simulink model "Three_Phase_Full_Wave_Uncontrolled_Rectifier"  (R2017b)
settings: Solver=VariableStepAuto  StartTime=0.0  StopTime=1.0  MaxStep=1e-4  RelTol=1e-3
libraries: powerlib x24, powerlib_meascontrol x5
settings Model: Creator=DELL  LastModifiedBy=DELL

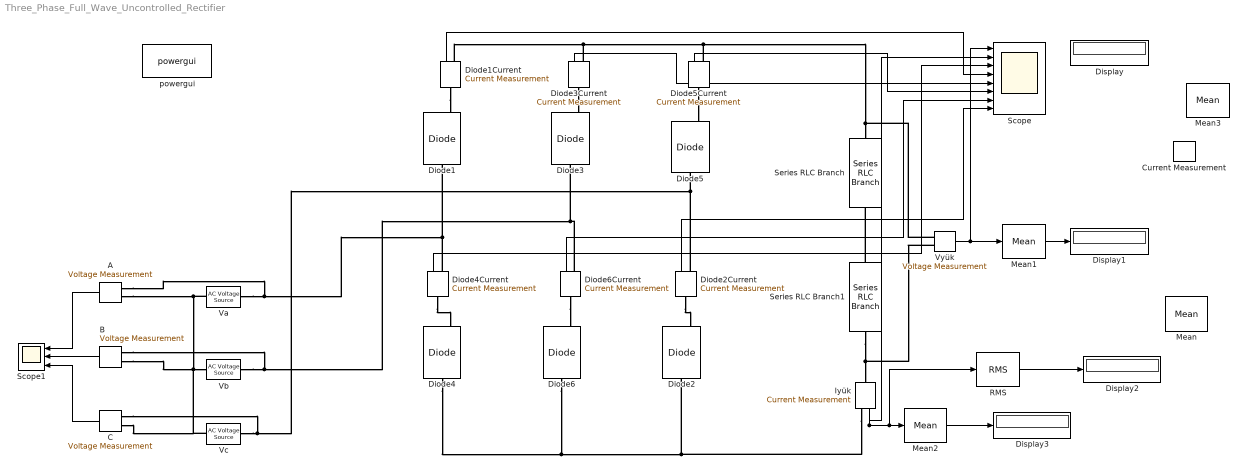
== system Three_Phase_Full_Wave_Uncontrolled_Rectifier ==
  A : powerlib/Measurements/Voltage Measurement  PhasorSimulation=off  OutputType=Complex  PSBequivalent=0
  B : powerlib/Measurements/Voltage Measurement  PhasorSimulation=off  OutputType=Complex  PSBequivalent=0
  C : powerlib/Measurements/Voltage Measurement  PhasorSimulation=off  OutputType=Complex  PSBequivalent=0
  Current Measurement : powerlib/Measurements/Current Measurement  PhasorSimulation=off  OutputType=Complex  PSBequivalent=0
  Diode{1..6} (6 alike) : powerlib/Power Electronics/Diode  Ron=0.001  Lon=0  Vf=0.8  IC=0  UseSnubber=0  Rs=500  Cs=250e-9  Measurements=on
  Diode1Current : powerlib/Measurements/Current Measurement  PhasorSimulation=off  OutputType=Complex  PSBequivalent=0
  Diode2Current : powerlib/Measurements/Current Measurement  PhasorSimulation=off  OutputType=Complex  PSBequivalent=0
  Diode3Current : powerlib/Measurements/Current Measurement  PhasorSimulation=off  OutputType=Complex  PSBequivalent=0
  Diode4Current : powerlib/Measurements/Current Measurement  PhasorSimulation=off  OutputType=Complex  PSBequivalent=0
  Diode5Current : powerlib/Measurements/Current Measurement  PhasorSimulation=off  OutputType=Complex  PSBequivalent=0
  Diode6Current : powerlib/Measurements/Current Measurement  PhasorSimulation=off  OutputType=Complex  PSBequivalent=0
  Display{,1..3} (4 alike) : Display
  Iyük : powerlib/Measurements/Current Measurement  PhasorSimulation=off  OutputType=Complex  PSBequivalent=0
  Mean : powerlib_meascontrol/Measurements/Mean  Freq=60  Vinit=0  Ts=0
  Mean1 : powerlib_meascontrol/Measurements/Mean  Freq=50  Vinit=0  Ts=0
  Mean2 : powerlib_meascontrol/Measurements/Mean  Freq=50  Vinit=0  Ts=0
  Mean3 : powerlib_meascontrol/Measurements/Mean  Freq=60  Vinit=0  Ts=0
  RMS : powerlib_meascontrol/Measurements/RMS  TrueRMS=on  Freq=50  RMSInit=120  Ts=0
  Scope : Scope  NumInputPorts=8
  Scope1 : Scope  NumInputPorts=3
  Series RLC Branch : powerlib/Elements/Series RLC Branch  LConnTagsString=__new0  RConnTagsString=__new0  BranchType=L  Resistance=1  Inductance=20e-3  SetiL0=off  InitialCurrent=0  Capacitance=1e-6  Setx0=off  InitialVoltage=0  Measurements=None
  Series RLC Branch1 : powerlib/Elements/Series RLC Branch  LConnTagsString=__new0  RConnTagsString=__new0  BranchType=R  Resistance=10  Inductance=1e-3  SetiL0=off  InitialCurrent=0  Capacitance=1e-6  Setx0=off  InitialVoltage=0  Measurements=None
  Va : powerlib/Electrical Sources/AC Voltage Source  Amplitude=220*(2^0.5)  Phase=0  Frequency=50  SampleTime=0  Measurements=None  BusType=swing  Pref=10e3  Qref=0  Qmin=-inf  Qmax=+inf
  Vb : powerlib/Electrical Sources/AC Voltage Source  Amplitude=220*(2^0.5)  Phase=-120  Frequency=50  SampleTime=0  Measurements=None  BusType=swing  Pref=10e3  Qref=0  Qmin=-inf  Qmax=+inf
  Vc : powerlib/Electrical Sources/AC Voltage Source  Amplitude=220*(2^0.5)  Phase=120  Frequency=50  SampleTime=0  Measurements=None  BusType=swing  Pref=10e3  Qref=0  Qmin=-inf  Qmax=+inf
  Vyük : powerlib/Measurements/Voltage Measurement  PhasorSimulation=off  OutputType=Complex  PSBequivalent=0
  powergui : powerlib/powergui  Priority=1  SimulationMode=Continuous  SampleTime=50e-6  frequency=60  Iterations=50  frequencyindice=50  Pbase=100e6  ErrMax=1e-4  UnitsV=kV  UnitsW=MW  buscounter=0  FunctionMessages=off  echomessages=off  EnableUseOfTLC=off  CurrentSourceSwitches=off  DisableSnubberDevices=off  DisableRonSwitches=off  DisableVfSwitches=off  DisplayEquations=off  SolverType=Tustin/Backward Euler (TBE)  Interpol=off  ExternalGateDelay=off  methode=off  Ts=100  x0status=blocks  SPID=on  SwTol=0  HookPort=off  RestoreLinks=warning  ResistiveCurrentMeasurement=off  Frange=[0:2:500]  Ylog=off  Xlog=on  ShowGrid=off  save=off  variable=ZData  structure=0  ZoomFFT=off  StartTime=0.0  cycles=1  DisplayStyle=1  fundamental=60  FreqAxis=off  MaxFrequency=1000  frequencyindicesteady=1  RmsSteady=1  display=off
  wires:
  A/1 -> Scope1/1
  B/1 -> Scope1/2
  C/1 -> Scope1/3
  Iyük/1 -> RMS/1, Mean2/1, Scope/2
  Vyük/1 -> Scope/1, Mean1/1
  Mean2/1 -> Display3/1
  RMS/1 -> Display2/1
  Mean1/1 -> Display1/1
  Diode5Current/1 -> Scope/6
  Diode4Current/1 -> Scope/3
  Diode1Current/1 -> Scope/4
  Diode3Current/1 -> Scope/5
  Diode6Current/1 -> Scope/7
  Diode2Current/1 -> Scope/8
  connections:
  Va/RConn1 -- A/LConn1 -- Diode4Current/RConn1 -- Diode1/LConn1
  Diode3Current/RConn1 -- Diode5Current/RConn1 -- Vyük/LConn1 -- Series RLC Branch/RConn1 -- Diode1Current/RConn1
  Series RLC Branch1/RConn1 -- Series RLC Branch/LConn1
  Diode6/LConn1 -- Iyük/RConn1 -- Diode2/LConn1 -- Diode4/LConn1
  Vb/RConn1 -- B/LConn1 -- Diode3/LConn1 -- Diode6Current/RConn1
  Vc/RConn1 -- C/LConn1 -- Diode5/LConn1 -- Diode2Current/RConn1
  Va/LConn1 -- Vc/LConn1 -- C/LConn2 -- B/LConn2 -- Vb/LConn1 -- A/LConn2
  Diode3Current/LConn1 -- Diode3/RConn1
  Diode1Current/LConn1 -- Diode1/RConn1
  Diode5Current/LConn1 -- Diode5/RConn1
  Series RLC Branch1/LConn1 -- Vyük/LConn2 -- Iyük/LConn1
  Diode4Current/LConn1 -- Diode4/RConn1
  Diode2Current/LConn1 -- Diode2/RConn1
  Diode6Current/LConn1 -- Diode6/RConn1
